simulink model "Model"  (R2020a)
settings: Solver=VariableStepAuto  StartTime=0.0  StopTime=10  RelTol=1e-3
undefined symbols (not defined in the file): b, d, g, I_b_bar, I_m_1_bar, I_m_2_bar, I_m_3_bar, I_m_4_bar, l, M, M_b, M_m, mu, Z_cg_0, Z_m_0
libraries: vrlib x4, sharedtransform x1, shared6dof x1, sharedutil x1, simulink x1
settings Model: Creator=Shahin  LastModifiedBy=Shahin

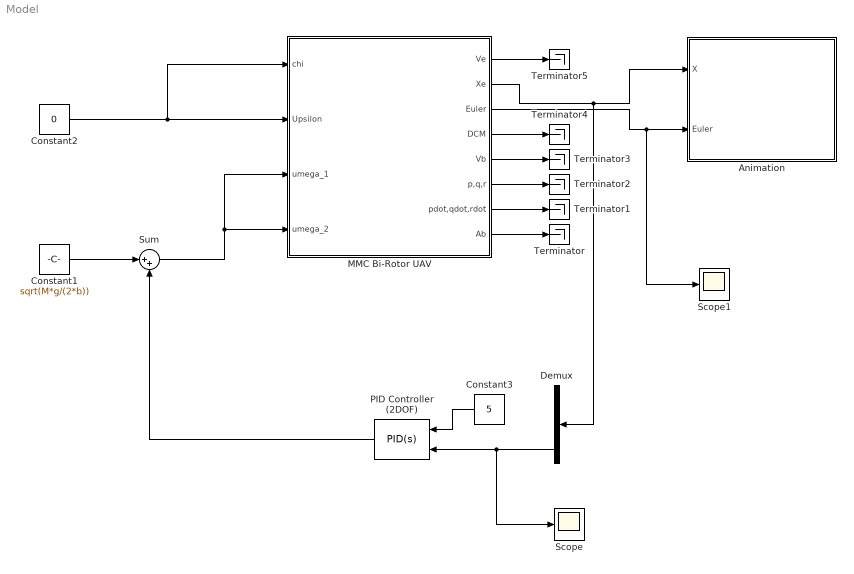
== system Model ==
  Animation : Subsystem
  Constant1 : Constant  Value=sqrt(M*g/(2*b))
  Constant2 : Constant  Value=0
  Constant3 : Constant  Value=5
  Demux : Demux  Outputs=3
  MMC Bi-Rotor UAV : Subsystem  InitFcn=|
      | %Initial Parameters
      | M_m          = 0.05;                                                           %MM mass
      | M_b           = 1.8;                                                             %Body mass
      | I_b_bar      = [0.1 0 0
      |                      0 0.1 0
      |                      0 0 0.01];                                                     %Inertia of the body around its CG
      | I_m_1_bar = [1 0 0
      |                     0 1 0
      |                     0 0 1].*1e-4;                                                 %Inertia of the MM1 around their CG
      | I_m_2_bar = [1 0 0
      |                     0 1 0
      |                     0 1 0].*1e-4;                                                 %Inertia of the MM2 around their CG
      | I_m_3_bar = [1 0 0
      |                     0 1 0
      |                     0 1 0].*1e-4;                                                 %Inertia of the MM3 around their CG
      | I_m_4_bar = [1 0 0
      |                     0 1 0
      |                     0 1 0].*1e-4;                                                 %Inertia of the MM4 around their CG
      | M              = M_b + 4*M_m;                                              %Total mass
      | mu            = M_m/M;                                                        %mass ratio
      | Z_b_0        = 0;                                                                 %z_cg body in R0
      | Z_m_0       = 0;                                                                 %z_cg MM in R0
      | Z_cg_0      = (Z_b_0*M_b + Z_m_0*M_m)/M;                      %z_cg total in R0
      | l                = 0.4;                                                             %max lenght of drone
      | b               = 0.00025;                                                          %Propeller thrust constant
      | d               = 0.000035;                                                        %Propeller drag constant
      | g               =9.81;                                                              %Gravity
  PID Controller (2DOF) : simulink/Continuous/PID Controller (2DOF)  Controller=PID  Form=Parallel  TimeDomain=Continuous-time  UseExternalTs=off  SampleTime=-1  IntegratorMethod=Forward Euler  FilterMethod=Forward Euler  ControllerParametersSource=internal  P=22.7153635435292  I=3.4696232596597  D=29.1878113477728  UseFilter=on  N=31.6784346154391  b=0.785342407546015  c=0.00291736985141084  TunerSelectOption=Transfer Function Based (PID Tuner App)  InitialConditionSource=internal  InitialConditionForIntegrator=0  InitialConditionForFilter=0  DifferentiatorICPrevScaledInput=0  ExternalReset=none  TrackingMode=off  Kt=1  LimitOutput=off  UpperSaturationLimit=inf  LowerSaturationLimit=-inf  LinearizeAsGain=on  AntiWindupMode=none  Kb=1  POutMin=[]  POutMax=[]  IOutMin=[]  IOutMax=[]  DOutMin=[]  DOutMax=[]  NOutMin=[]  NOutMax=[]  bOutMin=[]  bOutMax=[]  cOutMin=[]  cOutMax=[]  SumOutMin=[]  SumOutMax=[]  SaturationOutMin=[]  SaturationOutMax=[]  PParamMin=[]  PParamMax=[]  IParamMin=[]  IParamMax=[]  DParamMin=[]  DParamMax=[]  NParamMin=[]  NParamMax=[]  bParamMin=[]  bParamMax=[]  cParamMin=[]  cParamMax=[]  KbParamMin=[]  KbParamMax=[]  KtParamMin=[]  KtParamMax=[]  KbOutMin=[]  KbOutMax=[]  KtOutMin=[]  KtOutMax=[]  IntegratorOutMin=[]  IntegratorOutMax=[]  FilterOutMin=[]  FilterOutMax=[]  SumI1OutMin=[]  SumI1OutMax=[]  SumI2OutMin=[]  SumI2OutMax=[]  SumI3OutMin=[]  SumI3OutMax=[]  SumI4OutMin=[]  SumI4OutMax=[]  SumDOutMin=[]  SumDOutMax=[]  Sum1OutMin=[]  Sum1OutMax=[]  Sum2OutMin=[]  Sum2OutMax=[]  Sum3OutMin=[]  Sum3OutMax=[]  DifferentiatorOutMin=[]  DifferentiatorOutMax=[]  FilterDiffOutCoefMin=[]  FilterDiffOutCoefMax=[]  ReciprocalOutMin=[]  ReciprocalOutMax=[]  SumDenOutMin=[]  SumDenOutMax=[]  SumNumOutMin=[]  SumNumOutMax=[]  DivideOutMin=[]  DivideOutMax=[]  UdiffTsProdOutMin=[]  UdiffTsProdOutMax=[]  NTsProdOutMin=[]  NTsProdOutMax=[]  UintegralTsProdOutMin=[]  UintegralTsProdOutMax=[]  UngainTsProdOutMin=[]  UngainTsProdOutMax=[]  IntegratorContinuousStateAttributes=''  IntegratorStateMustResolveToSignalObject=off  IntegratorRTWStateStorageClass=Auto  FilterContinuousStateAttributes=''  FilterStateMustResolveToSignalObject=off  FilterRTWStateStorageClass=Auto  ParallelPVariant=InternalParameters  IdealPVariant=Disabled  IVariant=InternalParameters  DVariant=InternalParameters  bVariant=InternalParameters  cVariant=InternalParameters  IntegratorVariant=Continuous  SatVariant=Disabled  AWVariant=Passthrough  PCopyVariant=Disabled  TRVariant=Disabled  FdbkBlocksVariant=Forward  IdealPFdbkVariant=Disabled  SatFdbkVariant=Disabled  DerivativeFilterVariant=ContFilter  NVariant=InternalParameters  NCopyVariant=Disabled  FilterICVariant=InternalICsFilter  IntegratorICVariant=InternalICs  ExternalResetVariant=Disabled  TRSumVariant=Passthrough  SumFdbkVariant=Disabled  SumVariant=Sum_PID  TsampFilterVariant=InternalTs  TsampNgainVariant=Passthrough  TsampIntegralVariant=Passthrough
  Scope : Scope
  Scope1 : Scope
  Sum : Sum  Inputs=|++
  Terminator{,1..5} (6 alike) : Terminator
  wires:
  MMC Bi-Rotor UAV/8(Ab) -> Terminator/1
  MMC Bi-Rotor UAV/7(pdot,qdot,rdot) -> Terminator1/1
  MMC Bi-Rotor UAV/6(p,q,r) -> Terminator2/1
  MMC Bi-Rotor UAV/5(Vb) -> Terminator3/1
  MMC Bi-Rotor UAV/4(DCM) -> Terminator4/1
  MMC Bi-Rotor UAV/1(Ve) -> Terminator5/1
  Constant1/1 -> Sum/1
  Constant2/1 -> MMC Bi-Rotor UAV/1(chi), MMC Bi-Rotor UAV/2(Upsilon)
  MMC Bi-Rotor UAV/3(Euler) -> Scope1/1, Animation/2(Euler)
  MMC Bi-Rotor UAV/2(Xe) -> Demux/1, Animation/1(X)
  Demux/3 -> Scope/1, PID Controller (2DOF)/2
  Constant3/1 -> PID Controller (2DOF)/1
  PID Controller (2DOF)/1 -> Sum/2
  Sum/1 -> MMC Bi-Rotor UAV/4(umega_2), MMC Bi-Rotor UAV/3(umega_1)

== system Model/Animation ==
  X : Inport
  Euler : Inport  Port=2
  MATLAB to VR Coordinates : vrlib/Utilities/MATLAB to VR Coordinates
      settings: SourceProductBaseCode=SL
  Rotation Angles to Direction Cosine Matrix : sharedtransform/Rotation Angles to Direction Cosine Matrix  rotationOrder=XZY  aMode=aMode
      settings: SourceProductBaseCode=AE,PW,MT,VE,VP
  Rotation Matrix to VR Rotation : vrlib/Utilities/Rotation Matrix to VR Rotation  maxzero=1e-12
      settings: SourceProductBaseCode=SL
  VR Sink : vrlib/VR Sink  InstantiateOnLoad=on  SampleTime=0.1  ViewEnable=on  RemoteChange=off  RemoteView=off  FieldsWritten=drone.rotation.4.1.1.double#drone.translation.3.1.1.double  WorldFileName=vw.x3d  AutoView=off  VideoDimensions=[]  AllowVariableSize=off
  wires:
  Euler/1 -> Rotation Angles to Direction Cosine Matrix/1
  Rotation Matrix to VR Rotation/1 -> VR Sink/1
  Rotation Angles to Direction Cosine Matrix/1 -> Rotation Matrix to VR Rotation/1
  X/1 -> MATLAB to VR Coordinates/1
  MATLAB to VR Coordinates/1 -> VR Sink/2

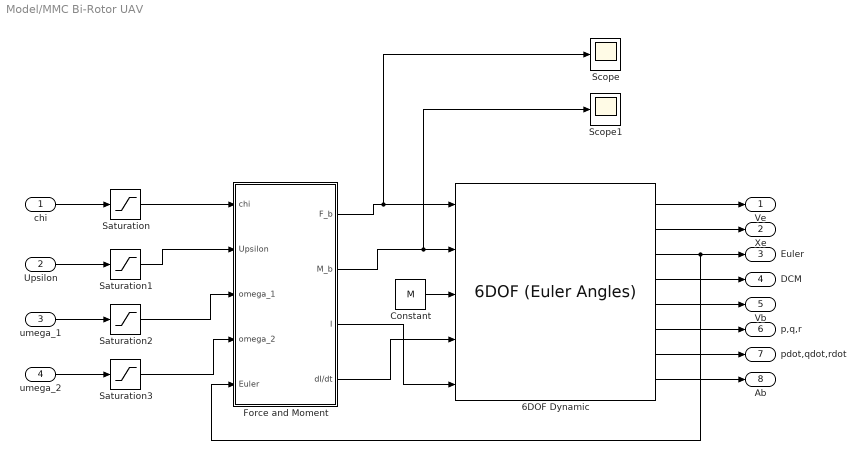
== system Model/MMC Bi-Rotor UAV ==
  chi : Inport
  Upsilon : Inport  Port=2
  umega_1 : Inport  Port=3
  umega_2 : Inport  Port=4
  6DOF Dynamic : shared6dof/6DOF (Euler Angles)  units=Metric (MKS)  mtype=Custom Variable  rep=Euler Angles  xme_0=[0 0 0]  Vm_0=[0 0 0]  eul_0=[0 0 0]  pm_0=[0 0 0]  mass_0=M  mass_e=0.5  mass_f=2.0  inertia=I  inertia_e=eye(3)  inertia_f=2*eye(3)  k_quat=1.0  vre_flag=off  abi_flag=off  aMode=0  xme_statename=''  Vm_statename=''  eul_statename=''  quat_statename=''  pm_statename=''  mass_statename=''
      settings: SourceProductBaseCode=AE,PW,MT,VE,VP
  Constant : Constant  Value=M
  Force and Moment : Subsystem
  Saturation : Saturate  UpperLimit=l/2  LowerLimit=-l/2
  Saturation1 : Saturate  UpperLimit=l/2  LowerLimit=-l/2
  Saturation2 : Saturate  UpperLimit=10000  LowerLimit=0
  Saturation3 : Saturate  UpperLimit=10000  LowerLimit=0
  Scope : Scope
  Scope1 : Scope
  Ve : Outport
  Xe : Outport  Port=2
  Euler : Outport  Port=3
  DCM : Outport  Port=4
  Vb : Outport  Port=5
  p,q,r : Outport  Port=6
  pdot,qdot,rdot : Outport  Port=7
  Ab : Outport  Port=8
  wires:
  6DOF Dynamic/4 -> DCM/1
  6DOF Dynamic/3 -> Force and Moment/5(Euler), Euler/1
  6DOF Dynamic/7 -> pdot,qdot,rdot/1
  6DOF Dynamic/8 -> Ab/1
  6DOF Dynamic/5 -> Vb/1
  6DOF Dynamic/1 -> Ve/1
  6DOF Dynamic/2 -> Xe/1
  6DOF Dynamic/6 -> p,q,r/1
  Force and Moment/1(F_b) -> Scope/1, 6DOF Dynamic/1
  Force and Moment/2(M_b) -> Scope1/1, 6DOF Dynamic/2
  chi/1 -> Saturation/1
  Upsilon/1 -> Saturation1/1
  umega_1/1 -> Saturation2/1
  umega_2/1 -> Saturation3/1
  Force and Moment/3(I) -> 6DOF Dynamic/5
  Force and Moment/4(dI/dt) -> 6DOF Dynamic/4
  Constant/1 -> 6DOF Dynamic/3
  Saturation/1 -> Force and Moment/1(chi)
  Saturation1/1 -> Force and Moment/2(Upsilon)
  Saturation2/1 -> Force and Moment/3(omega_1)
  Saturation3/1 -> Force and Moment/4(omega_2)

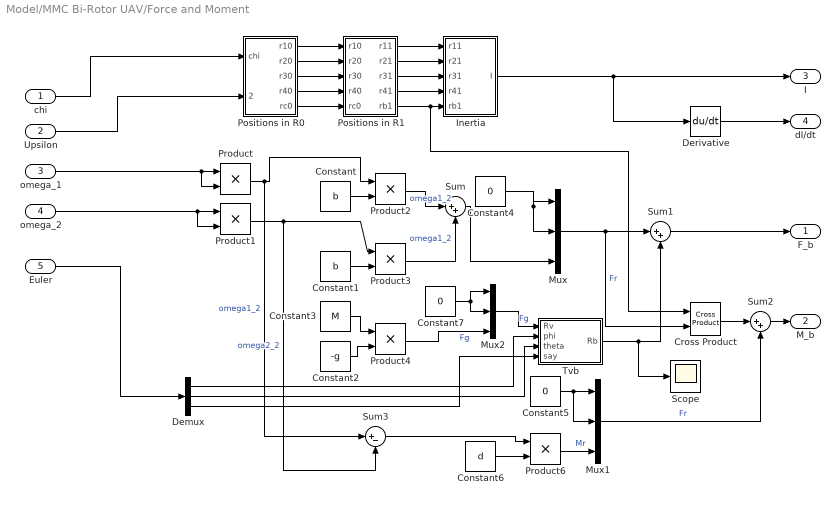
== system Model/MMC Bi-Rotor UAV/Force and Moment ==
  chi : Inport
  Upsilon : Inport  Port=2
  omega_1 : Inport  Port=3
  omega_2 : Inport  Port=4
  Euler : Inport  Port=5
  Constant : Constant  Value=b
  Constant1 : Constant  Value=b
  Constant2 : Constant  Value=-g
  Constant3 : Constant  Value=M
  Constant4 : Constant  Value=0
  Constant5 : Constant  Value=0
  Constant6 : Constant  Value=d
  Constant7 : Constant  Value=0
  Cross Product : vrlib/Utilities/Cross Product
  Demux : Demux  Outputs=3
  Derivative : Derivative
  Inertia : Subsystem
  Mux : Mux  Inputs=3
  Mux1 : Mux  Inputs=3
  Mux2 : Mux  Inputs=3
  Positions in R0 : Subsystem
  Positions in R1 : Subsystem
  Product{,1..4,6} (6 alike) : Product
  Scope : Scope
  Sum : Sum  Inputs=|++
  Sum1 : Sum  Inputs=|++
  Sum2 : Sum  Inputs=|++
  Sum3 : Sum  Inputs=|+-
  Tvb : Subsystem
  F_b : Outport
  M_b : Outport  Port=2
  I : Outport  Port=3
  dI/dt : Outport  Port=4
  wires:
  chi/1 -> Positions in R0/1(chi)
  Upsilon/1 -> Positions in R0/2(Upsilon)
  Positions in R0/1(r10) -> Positions in R1/1(r10)
  Positions in R0/2(r20) -> Positions in R1/2(r20)
  Positions in R0/3(r30) -> Positions in R1/3(r30)
  Positions in R0/4(r40) -> Positions in R1/4(r40)
  Positions in R0/5(rc0) -> Positions in R1/5(rc0)
  Positions in R1/1(r11) -> Inertia/1(r11)
  Positions in R1/2(r21) -> Inertia/2(r21)
  Positions in R1/3(r31) -> Inertia/3(r31)
  Positions in R1/4(r41) -> Inertia/4(r41)
  Positions in R1/5(rb1) -> Cross Product/1, Inertia/5(rb1)
  omega_1/1 -> Product/2, Product/1
  Product/1 -> Sum3/1, Product2/1  "omega1_2"
  omega_2/1 -> Product1/2, Product1/1
  Product1/1 -> Sum3/2, Product3/1  "omega2_2"
  Constant/1 -> Product2/2
  Constant1/1 -> Product3/2
  Constant2/1 -> Product4/2
  Constant3/1 -> Product4/1
  Product2/1 -> Sum/1  "omega1_2"
  Product3/1 -> Sum/2  "omega1_2"
  Sum/1 -> Mux/3
  Constant4/1 -> Mux/2, Mux/1
  Mux/1 -> Cross Product/2, Sum1/1  "Fr"
  Sum1/1 -> F_b/1
  Tvb/1(Rb) -> Scope/1, Sum1/2
  Euler/1 -> Demux/1
  Demux/1 -> Tvb/2(phi)
  Demux/2 -> Tvb/3(theta)
  Demux/3 -> Tvb/4(say)
  Sum2/1 -> M_b/1
  Cross Product/1 -> Sum2/1
  Mux1/1 -> Sum2/2  "Fr"
  Constant5/1 -> Mux1/2, Mux1/1
  Product6/1 -> Mux1/3  "Mr"
  Sum3/1 -> Product6/1
  Constant6/1 -> Product6/2
  Derivative/1 -> dI/dt/1
  Inertia/1(I) -> Derivative/1, I/1
  Product4/1 -> Mux2/3  "Fg"
  Mux2/1 -> Tvb/1(Rv)  "Fg"
  Constant7/1 -> Mux2/1, Mux2/2

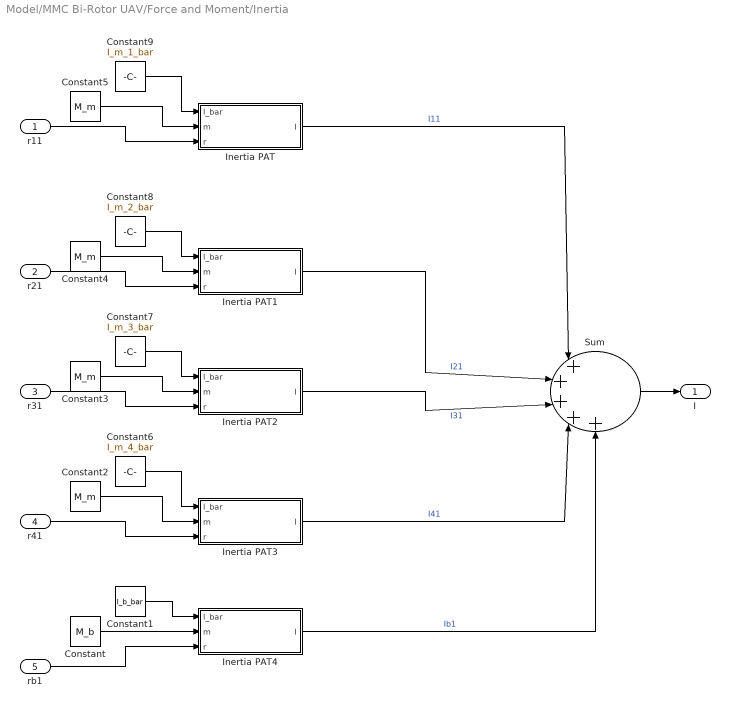
== system Model/MMC Bi-Rotor UAV/Force and Moment/Inertia ==
  r11 : Inport
  r21 : Inport  Port=2
  r31 : Inport  Port=3
  r41 : Inport  Port=4
  rb1 : Inport  Port=5
  Constant : Constant  Value=M_b
  Constant1 : Constant  Value=I_b_bar
  Constant{2..5} (4 alike) : Constant  Value=M_m
  Constant6 : Constant  Value=I_m_4_bar
  Constant7 : Constant  Value=I_m_3_bar
  Constant8 : Constant  Value=I_m_2_bar
  Constant9 : Constant  Value=I_m_1_bar
  Inertia PAT : Subsystem
  Inertia PAT1 : Subsystem
  Inertia PAT2 : Subsystem
  Inertia PAT3 : Subsystem
  Inertia PAT4 : Subsystem
  Sum : Sum  Inputs=|+++++
  I : Outport
  wires:
  Inertia PAT1/1(I) -> Sum/2  "I21"
  Inertia PAT2/1(I) -> Sum/3  "I31"
  Inertia PAT3/1(I) -> Sum/4  "I41"
  Inertia PAT4/1(I) -> Sum/5  "Ib1"
  r11/1 -> Inertia PAT/3(r)
  r21/1 -> Inertia PAT1/3(r)
  r31/1 -> Inertia PAT2/3(r)
  r41/1 -> Inertia PAT3/3(r)
  rb1/1 -> Inertia PAT4/3(r)
  Constant/1 -> Inertia PAT4/2(m)
  Constant1/1 -> Inertia PAT4/1(I_bar)
  Constant2/1 -> Inertia PAT3/2(m)
  Constant3/1 -> Inertia PAT2/2(m)
  Constant4/1 -> Inertia PAT1/2(m)
  Constant5/1 -> Inertia PAT/2(m)
  Constant6/1 -> Inertia PAT3/1(I_bar)
  Constant7/1 -> Inertia PAT2/1(I_bar)
  Constant8/1 -> Inertia PAT1/1(I_bar)
  Constant9/1 -> Inertia PAT/1(I_bar)
  Inertia PAT/1(I) -> Sum/1  "I11"
  Sum/1 -> I/1

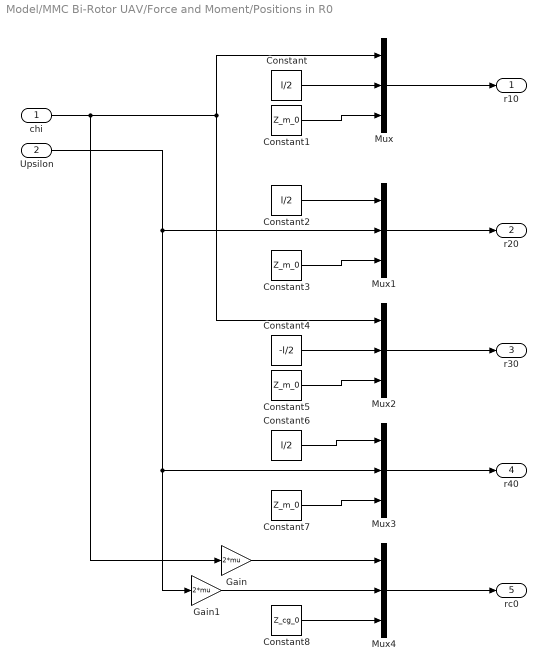
== system Model/MMC Bi-Rotor UAV/Force and Moment/Positions in R0 ==
  chi : Inport
  Upsilon : Inport  Port=2
  Constant : Constant  Value=l/2
  Constant{1,3,5,7} (4 alike) : Constant  Value=Z_m_0
  Constant2 : Constant  Value=l/2
  Constant4 : Constant  Value=-l/2
  Constant6 : Constant  Value=l/2
  Constant8 : Constant  Value=Z_cg_0
  Gain : Gain  Gain=2*mu
  Gain1 : Gain  Gain=2*mu
  Mux{,1..4} (5 alike) : Mux  Inputs=3
  r10 : Outport
  r20 : Outport  Port=2
  r30 : Outport  Port=3
  r40 : Outport  Port=4
  rc0 : Outport  Port=5
  wires:
  Constant/1 -> Mux/2
  Constant1/1 -> Mux/3
  Mux/1 -> r10/1
  Mux1/1 -> r20/1
  Constant3/1 -> Mux1/3
  Constant2/1 -> Mux1/1
  Constant4/1 -> Mux2/2
  Constant5/1 -> Mux2/3
  Mux2/1 -> r30/1
  Mux3/1 -> r40/1
  Constant7/1 -> Mux3/3
  Constant6/1 -> Mux3/1
  Upsilon/1 -> Mux3/2, Gain1/1, Mux1/2
  Mux4/1 -> rc0/1
  Constant8/1 -> Mux4/3
  chi/1 -> Gain/1, Mux/1, Mux2/1
  Gain/1 -> Mux4/1
  Gain1/1 -> Mux4/2

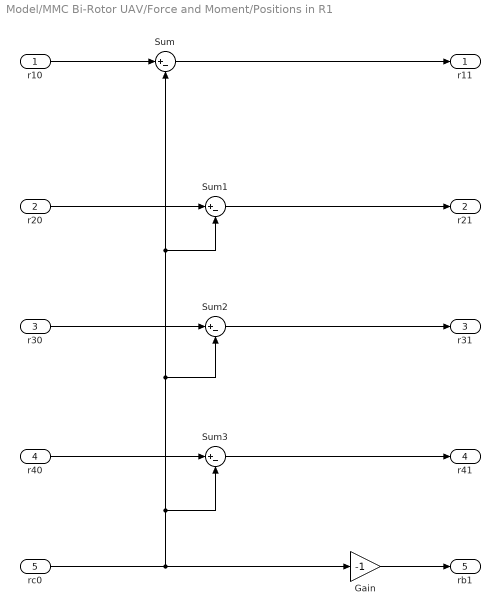
== system Model/MMC Bi-Rotor UAV/Force and Moment/Positions in R1 ==
  r10 : Inport
  r20 : Inport  Port=2
  r30 : Inport  Port=3
  r40 : Inport  Port=4
  rc0 : Inport  Port=5
  Gain : Gain  Gain=-1
  Sum{,1..3} (4 alike) : Sum  Inputs=|+-
  r11 : Outport
  r21 : Outport  Port=2
  r31 : Outport  Port=3
  r41 : Outport  Port=4
  rb1 : Outport  Port=5
  wires:
  r10/1 -> Sum/1
  rc0/1 -> Gain/1, Sum3/2, Sum2/2, Sum1/2, Sum/2
  Sum/1 -> r11/1
  r20/1 -> Sum1/1
  Sum1/1 -> r21/1
  Sum2/1 -> r31/1
  r30/1 -> Sum2/1
  r40/1 -> Sum3/1
  Sum3/1 -> r41/1
  Gain/1 -> rb1/1

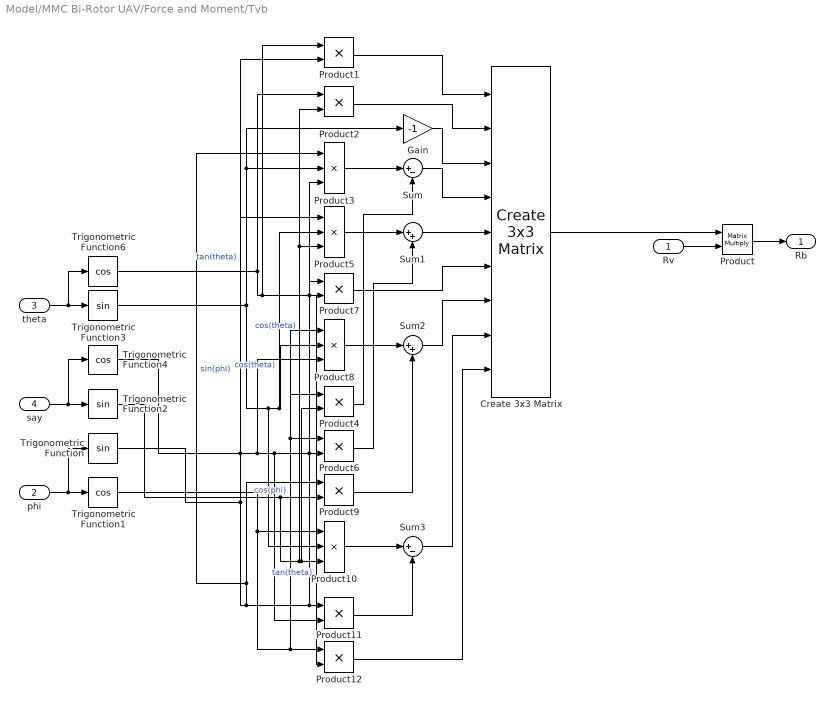
== system Model/MMC Bi-Rotor UAV/Force and Moment/Tvb ==
  Rv : Inport
  phi : Inport  Port=2
  theta : Inport  Port=3
  say : Inport  Port=4
  Create 3x3 Matrix : sharedutil/Create 3x3 Matrix  aMode=aMode
      settings: SourceProductBaseCode=AE,PW,MT,VE,VP
  Gain : Gain  Gain=-1
  Product : Product  Multiplication=Matrix(*)
  Product{1..2,4,6..7,9,11..12} (8 alike) : Product
  Product{3,5,8,10} (4 alike) : Product  Inputs=3
  Sum : Sum  Inputs=|+-
  Sum1 : Sum  Inputs=|++
  Sum2 : Sum  Inputs=|++
  Sum3 : Sum  Inputs=|+-
  Trigonometric Function : Trigonometry
  Trigonometric Function1 : Trigonometry  Operator=cos
  Trigonometric Function2 : Trigonometry
  Trigonometric Function3 : Trigonometry
  Trigonometric Function4 : Trigonometry  Operator=cos
  Trigonometric Function6 : Trigonometry  Operator=cos
  Rb : Outport
  wires:
  Product2/1 -> Create 3x3 Matrix/2
  Sum1/1 -> Create 3x3 Matrix/5
  Product5/1 -> Sum1/1
  Create 3x3 Matrix/1 -> Product/1
  Trigonometric Function4/1 -> Product6/2, Product3/3, Product11/2, Product8/3, Product1/2  "tan(theta)"
  Product/1 -> Rb/1
  Rv/1 -> Product/2
  Product1/1 -> Create 3x3 Matrix/1
  Sum/1 -> Create 3x3 Matrix/4
  Gain/1 -> Create 3x3 Matrix/3
  Product4/1 -> Sum/2
  Product3/1 -> Sum/1
  Product7/1 -> Create 3x3 Matrix/6
  Sum2/1 -> Create 3x3 Matrix/7
  say/1 -> Trigonometric Function2/1, Trigonometric Function4/1
  Product8/1 -> Sum2/1
  Sum3/1 -> Create 3x3 Matrix/8
  phi/1 -> Trigonometric Function/1, Trigonometric Function1/1
  Product10/1 -> Sum3/1
  Product6/1 -> Sum1/2
  theta/1 -> Trigonometric Function3/1, Trigonometric Function6/1
  Product11/1 -> Sum3/2
  Product12/1 -> Create 3x3 Matrix/9
  Product9/1 -> Sum2/2
  Trigonometric Function6/1 -> Product2/1, Product12/2, Product7/2, Product1/1  "tan(theta)"
  Trigonometric Function2/1 -> Product10/3, Product4/2, Product5/3, Product2/2, Product9/2  "cos(theta)"
  Trigonometric Function3/1 -> Product8/2, Product5/2, Product10/2, Gain/1, Product3/2  "cos(theta)"
  Trigonometric Function/1 -> Product11/1, Product7/1, Product9/1, Product3/1, Product5/1  "sin(phi)"
  Trigonometric Function1/1 -> Product4/1, Product6/1, Product12/1, Product8/1, Product10/1  "cos(phi)"

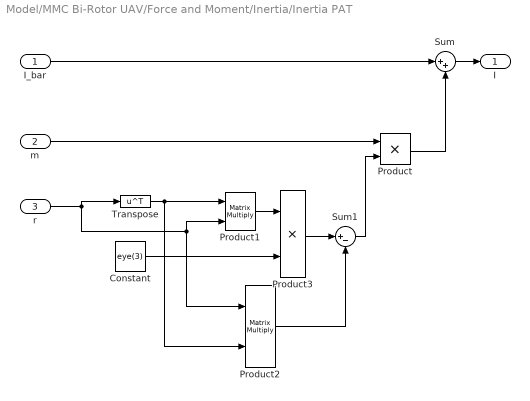
== system Model/MMC Bi-Rotor UAV/Force and Moment/Inertia/Inertia PAT ==
  I_bar : Inport
  m : Inport  Port=2
  r : Inport  Port=3
  Constant : Constant  Value=eye(3)
  Product : Product
  Product1 : Product  Multiplication=Matrix(*)
  Product2 : Product  Multiplication=Matrix(*)
  Product3 : Product
  Sum : Sum  Inputs=|++
  Sum1 : Sum  Inputs=|+-
  Transpose : Math  Operator=transpose  SaturateOnIntegerOverflow=on
  I : Outport
  wires:
  I_bar/1 -> Sum/1
  Sum/1 -> I/1
  m/1 -> Product/1
  Product/1 -> Sum/2
  r/1 -> Transpose/1, Product2/1, Product1/2
  Transpose/1 -> Product2/2, Product1/1
  Constant/1 -> Product3/2
  Product1/1 -> Product3/1
  Product2/1 -> Sum1/2
  Sum1/1 -> Product/2
  Product3/1 -> Sum1/1

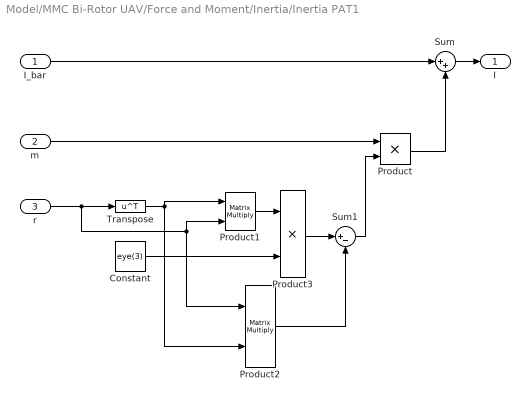
== system Model/MMC Bi-Rotor UAV/Force and Moment/Inertia/Inertia PAT1 ==
  I_bar : Inport
  m : Inport  Port=2
  r : Inport  Port=3
  Constant : Constant  Value=eye(3)
  Product : Product
  Product1 : Product  Multiplication=Matrix(*)
  Product2 : Product  Multiplication=Matrix(*)
  Product3 : Product
  Sum : Sum  Inputs=|++
  Sum1 : Sum  Inputs=|+-
  Transpose : Math  Operator=transpose  SaturateOnIntegerOverflow=on
  I : Outport
  wires:
  Product3/1 -> Sum1/1
  Sum1/1 -> Product/2
  Product2/1 -> Sum1/2
  Product1/1 -> Product3/1
  Constant/1 -> Product3/2
  Transpose/1 -> Product1/1, Product2/2
  r/1 -> Transpose/1, Product1/2, Product2/1
  Product/1 -> Sum/2
  m/1 -> Product/1
  Sum/1 -> I/1
  I_bar/1 -> Sum/1

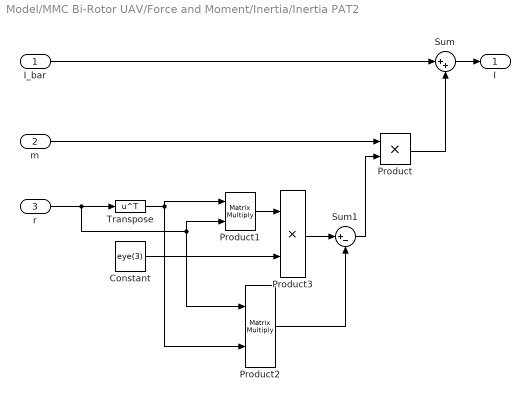
== system Model/MMC Bi-Rotor UAV/Force and Moment/Inertia/Inertia PAT2 ==
  I_bar : Inport
  m : Inport  Port=2
  r : Inport  Port=3
  Constant : Constant  Value=eye(3)
  Product : Product
  Product1 : Product  Multiplication=Matrix(*)
  Product2 : Product  Multiplication=Matrix(*)
  Product3 : Product
  Sum : Sum  Inputs=|++
  Sum1 : Sum  Inputs=|+-
  Transpose : Math  Operator=transpose  SaturateOnIntegerOverflow=on
  I : Outport
  wires:
  I_bar/1 -> Sum/1
  Sum/1 -> I/1
  m/1 -> Product/1
  Product/1 -> Sum/2
  r/1 -> Transpose/1, Product2/1, Product1/2
  Transpose/1 -> Product2/2, Product1/1
  Constant/1 -> Product3/2
  Product1/1 -> Product3/1
  Product2/1 -> Sum1/2
  Sum1/1 -> Product/2
  Product3/1 -> Sum1/1

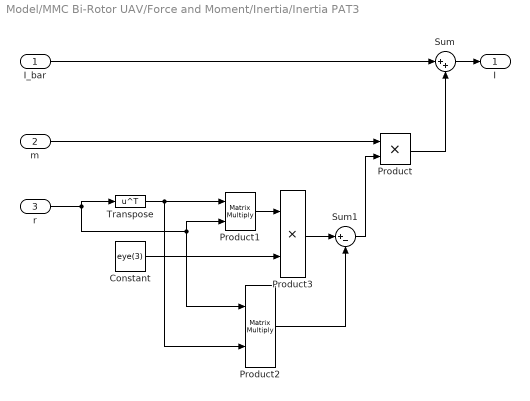
== system Model/MMC Bi-Rotor UAV/Force and Moment/Inertia/Inertia PAT3 ==
  I_bar : Inport
  m : Inport  Port=2
  r : Inport  Port=3
  Constant : Constant  Value=eye(3)
  Product : Product
  Product1 : Product  Multiplication=Matrix(*)
  Product2 : Product  Multiplication=Matrix(*)
  Product3 : Product
  Sum : Sum  Inputs=|++
  Sum1 : Sum  Inputs=|+-
  Transpose : Math  Operator=transpose  SaturateOnIntegerOverflow=on
  I : Outport
  wires:
  Product3/1 -> Sum1/1
  Sum1/1 -> Product/2
  Product2/1 -> Sum1/2
  Product1/1 -> Product3/1
  Constant/1 -> Product3/2
  Transpose/1 -> Product2/2, Product1/1
  r/1 -> Transpose/1, Product1/2, Product2/1
  Product/1 -> Sum/2
  m/1 -> Product/1
  Sum/1 -> I/1
  I_bar/1 -> Sum/1

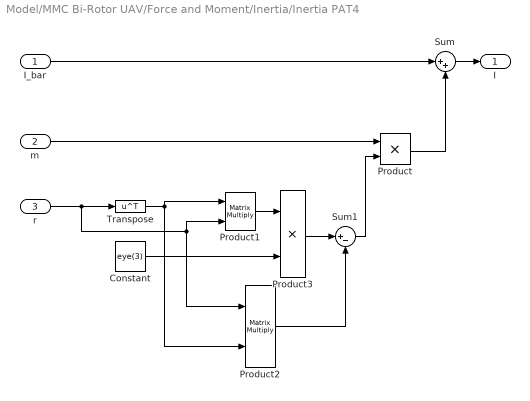
== system Model/MMC Bi-Rotor UAV/Force and Moment/Inertia/Inertia PAT4 ==
  I_bar : Inport
  m : Inport  Port=2
  r : Inport  Port=3
  Constant : Constant  Value=eye(3)
  Product : Product
  Product1 : Product  Multiplication=Matrix(*)
  Product2 : Product  Multiplication=Matrix(*)
  Product3 : Product
  Sum : Sum  Inputs=|++
  Sum1 : Sum  Inputs=|+-
  Transpose : Math  Operator=transpose  SaturateOnIntegerOverflow=on
  I : Outport
  wires:
  I_bar/1 -> Sum/1
  Sum/1 -> I/1
  m/1 -> Product/1
  Product/1 -> Sum/2
  r/1 -> Transpose/1, Product2/1, Product1/2
  Transpose/1 -> Product2/2, Product1/1
  Constant/1 -> Product3/2
  Product1/1 -> Product3/1
  Product2/1 -> Sum1/2
  Sum1/1 -> Product/2
  Product3/1 -> Sum1/1
